simulink model " PV_PEM_direct"  (R2026a)
settings: Solver=VariableStepAuto  StopTime=sim_t
values from neighbouring files (symbols this model uses):
  Active_Area = 17.64    [ PV_PEM_direct.m]    (also in PV_PEM_direct.m)
  Irr_stair_time = (0 : Irr_stair_tsamp : sim_t)'    [ PV_PEM_direct.m]    (also in PV_PEM_direct.m)
  Irr_stair_val = interp1(Irr_time, Irr_val,  Irr_stair_time, 'linear', 0)    [ PV_PEM_direct.m]    (also in PV_PEM_direct.m)
  N = 13    [ PV_PEM_direct.m]    (also in PV_PEM_direct.m = 16)
  Ra_stack = Ra   * N    (= 0.02301)    [ PV_PEM_direct.m]    (also in PV_PEM_direct.m = 0.02832)
  Rc_stack = Rc   * N    (= 0.0065)    [ PV_PEM_direct.m]    (also in PV_PEM_direct.m = 0.008)
  Rint_stack = Rint * N    (= 0.112749)    [ PV_PEM_direct.m]    (also in PV_PEM_direct.m = 0.138768)
  sample_output_time = 60 / scale_factor    (= 0.00166666666667)    [ PV_PEM_direct.m]    (also in PV_PEM_direct.m)
  Vint_stack = Vint * N    (= 19.185933)    [ PV_PEM_direct.m]    (also in PV_PEM_direct.m = 23.613456)
libraries: fl_lib x14, nesl_utility x9, simulink x1, ee_lib x1
settings Model: Creator=hanna  LastModifiedBy=Diamantis
settings SimscapeCC: SimscapeNominalValues="[{\"value\":\"1\",\"unit\":\"A\"},{\"value\":\"1\",\"unit\":\"bar\"},{\"value\":\"1\",\"unit\":\"cm^2\"},{\"value\":\"1\",\"unit\":\"cm^3/s\"},{\"value\":\"1\",\"unit\":\"kJ/kg\"},{\"value\":\"1\",\"unit\":\"kW\"},{\"value\":\"1\",\"unit\":\"l\"},{\"value\":\"1\",\"unit\":\"N\"},{\"value\":\"1\",\"unit\":\"N*m\"},{\"value\":\"1\",\"unit\":\"V\"}]"  SimscapeLogType=none  SimscapeLogDataHistory=5000.0

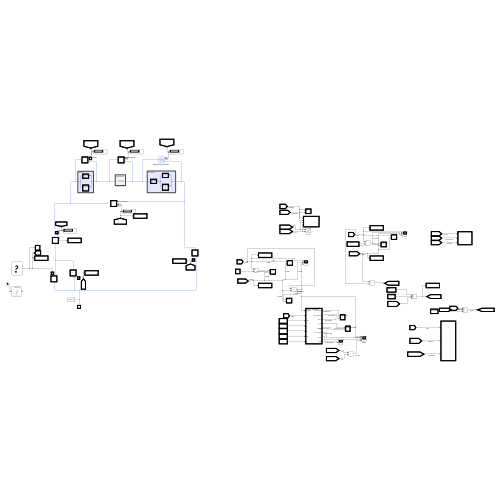
[thumbnail: Simulink's stored preview of the top-level diagram]
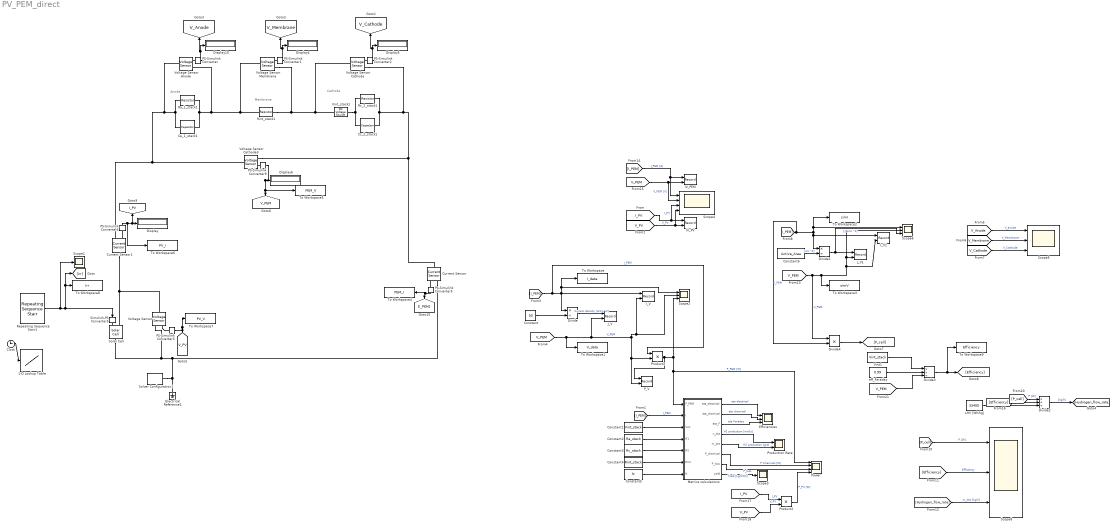
== system  PV_PEM_direct ==
  note: Membrane
  note: Cathode
  note: Anode
  1-D Lookup Table : Lookup_n-D  NumberOfTableDimensions=1  BreakpointsForDimension1=Irr_stair_time  Table=Irr_stair_val  InternalRulePriority=Speed  RndMeth=Simplest
  Ca_1_stack1 : fl_lib/Electrical/Electrical Elements/Capacitor  c=Ca_stack F  r=1e-6 Ohm  g=0 1/Ohm  i_specify=off  i_priority=None  i=0 A  i_nominal_specify=off  i_nominal_value=1  i_nominal_unit=A  v_specify=off  v_priority=None  v=0 V  v_nominal_specify=off  v_nominal_value=1  v_nominal_unit=V  vc_specify=off  vc_priority=High  vc=0 V  vc_nominal_specify=off  vc_nominal_value=1  vc_nominal_unit=V
  Cc_2_stack1 : fl_lib/Electrical/Electrical Elements/Capacitor  c=Cc_stack F  r=1e-6 Ohm  g=0 1/Ohm  i_specify=off  i_priority=None  i=0 A  i_nominal_specify=off  i_nominal_value=1  i_nominal_unit=A  v_specify=off  v_priority=None  v=0 V  v_nominal_specify=off  v_nominal_value=1  v_nominal_unit=V  vc_specify=off  vc_priority=High  vc=0 V  vc_nominal_specify=off  vc_nominal_value=1  vc_nominal_unit=V
  Clock : Clock
  Constant : Constant  Value=50
  Constant1 : Constant  Value=Vint_stack
  Constant2 : Constant  Value=Ra_stack
  Constant3 : Constant  Value=Rc_stack
  Constant4 : Constant  Value=Rint_stack
  Constant5 : Constant  Value=N
  Constant6 : Constant  Value=Active_Area
  Current Sensor : fl_lib/Electrical/Electrical Sensors/Current Sensor
  Current Sensor1 : fl_lib/Electrical/Electrical Sensors/Current Sensor
  Display{,4..6,10} (5 alike) : Display
  Divide : Product  Inputs=*/
  Divide1 : Product  Inputs=*/
  Divide2 : Product  Inputs=**/
  Divide3 : Product  Inputs=**/
  Divide4 : Product  Inputs=**
  Efficiencies : Scope  NumInputPorts=3
      settings: ActiveDisplayYMinimum=-1  ActiveDisplayYMaximum=1  DataLoggingVariableName=ScopeData5
  Electrical Reference1 : fl_lib/Electrical/Electrical Elements/Electrical Reference
  IV_PEM : Record  NumPorts=2.0  FileSettingsInternal="{\"entries\":[{\"content\":{\"excelSettings\":{\"content\":{},\"type\":\"Streamout.ExcelSettings\"},\"parquetSettings\":{\"content\":{},\"type\":\"Streamout.ParquetSettings\"}},\"type\":\"Streamout.FileSettingStorage\",\"uuid\":\"\"}],\"packageUris\":[\"http:\\/\\/schema.mathworks.com\\/mf0\\/streamout_blocks\\/R2020a\"],\"version\":\"1.0\"}"  FrameSettings=[0, 0]  Layout=[1 1]  SignalsInternal="{\"entries\":[{\"content\":{\"signals\":[{\"content\":{\"blockPath\":[],\"dimensions\":[1],\"domain\":\"\",\"lineColor\":\"#edb120\",\"lineWidth\":2,\"port\":1,\"signalID\":1,\"signalName\":\"I_PEM [A]\"},\"type\":\"RecordBlkView.Signal\",\"uuid\":\"\"},{\"content\":{\"blockPath\":[],\"dimensions\":[1],\"domain\":\"\",\"lineColor\":\"#7e2f8e\",\"lineWidth\":2,\"port\":2,\"signalID\":2,\"signalName\":\"V_PEM [V]\"},\"type\":\"RecordBlkView.Signal\",\"uuid\":\"\"}]},\"type\":\"RecordBlkView.InputSignals\",\"uuid\":\"\"}],\"packageUris\":[\"http:\\/\\/schema.mathworks.com\\/mf0\\/streamout_blocks\\/R2020a\"],\"version\":\"1.0\"}"  VisualizationBindings="{\"xyplotplugin\":{\"info\":[{\"series\":[],\"subplotID\":1}]}}"  CompatibilityTag=XY
  IV_PV : Record  NumPorts=2.0  FileSettingsInternal="{\"entries\":[{\"content\":{\"excelSettings\":{\"content\":{},\"type\":\"Streamout.ExcelSettings\"},\"parquetSettings\":{\"content\":{},\"type\":\"Streamout.ParquetSettings\"}},\"type\":\"Streamout.FileSettingStorage\",\"uuid\":\"\"}],\"packageUris\":[\"http:\\/\\/schema.mathworks.com\\/mf0\\/streamout_blocks\\/R2020a\"],\"version\":\"1.0\"}"  FrameSettings=[0, 0]  Layout=[1 1]  SignalsInternal="{\"entries\":[{\"content\":{\"signals\":[{\"content\":{\"blockPath\":[],\"dimensions\":[1],\"domain\":\"\",\"lineColor\":\"#a2142f\",\"plots\":[ 1 ],\"port\":1,\"signalID\":1,\"signalName\":\"I_PV\"},\"type\":\"RecordBlkView.Signal\",\"uuid\":\"\"},{\"content\":{\"blockPath\":[],\"dimensions\":[1],\"domain\":\"\",\"lineColor\":\"#139fff\",\"plots\":[ 1 ],\"port\":2,\"signalID\":2,\"signalName\":\"V_PV\"},\"type\":\"RecordBlkView.Signal\",\"uuid\":\"\"}]},\"type\":\"RecordBlkView.InputSignals\",\"uuid\":\"\"}],\"packageUris\":[\"http:\\/\\/schema.mathworks.com\\/mf0\\/streamout_blocks\\/R2020a\"],\"version\":\"1.0\"}"  VisualizationBindings="{\"xyplotplugin\":{\"info\":[{\"series\":[{\"bindingParametersList\":[{\"parameter\":\"X-Axis\",\"signalID\":1,\"signalName\":\"I_PV\"},{\"parameter\":\"Y-Axis\",\"signalID\":2,\"signalName\":\"V_PV\"}],\"seriesID\":0}],\"subplotID\":1}]}}"  CompatibilityTag=XY
  I_V : Record  NumPorts=2.0  FileSettingsInternal="{\"entries\":[{\"content\":{\"excelSettings\":{\"content\":{},\"type\":\"Streamout.ExcelSettings\"},\"parquetSettings\":{\"content\":{},\"type\":\"Streamout.ParquetSettings\"}},\"type\":\"Streamout.FileSettingStorage\",\"uuid\":\"\"}],\"packageUris\":[\"http:\\/\\/schema.mathworks.com\\/mf0\\/streamout_blocks\\/R2020a\"],\"version\":\"1.0\"}"  FrameSettings=[0, 0]  Layout=[1 1]  SignalsInternal="{\"entries\":[{\"content\":{\"signals\":[{\"content\":{\"blockPath\":[],\"dimensions\":[1],\"domain\":\"\",\"lineColor\":\"#a2142f\",\"lineWidth\":2,\"port\":1,\"signalID\":1,\"signalName\":\"I_PEM\"},\"type\":\"RecordBlkView.Signal\",\"uuid\":\"\"},{\"content\":{\"blockPath\":[],\"dimensions\":[1],\"domain\":\"\",\"lineColor\":\"#139fff\",\"lineWidth\":2,\"port\":2,\"signalID\":2,\"signalName\":\"V_PEM\"},\"type\":\"RecordBlkView.Signal\",\"uuid\":\"\"}]},\"type\":\"RecordBlkView.InputSignals\",\"uuid\":\"\"}],\"packageUris\":[\"http:\\/\\/schema.mathworks.com\\/mf0\\/streamout_blocks\\/R2020a\"],\"version\":\"1.0\"}"  VisualizationBindings="{\"xyplotplugin\":{\"info\":[{\"series\":[],\"subplotID\":1}]}}"  CompatibilityTag=XY
  I_V1 : Record  NumPorts=2.0  FileSettingsInternal="{\"entries\":[{\"content\":{\"excelSettings\":{\"content\":{},\"type\":\"Streamout.ExcelSettings\"},\"parquetSettings\":{\"content\":{},\"type\":\"Streamout.ParquetSettings\"}},\"type\":\"Streamout.FileSettingStorage\",\"uuid\":\"\"}],\"packageUris\":[\"http:\\/\\/schema.mathworks.com\\/mf0\\/streamout_blocks\\/R2020a\"],\"version\":\"1.0\"}"  FrameSettings=[0, 0]  Layout=[1 1]  SignalsInternal="{\"entries\":[{\"content\":{\"signals\":[{\"content\":{\"blockPath\":[],\"dimensions\":[1],\"domain\":\"\",\"lineColor\":\"#ff6929\",\"lineWidth\":2,\"port\":1,\"signalID\":1,\"signalName\":\"I_PEM\"},\"type\":\"RecordBlkView.Signal\",\"uuid\":\"\"},{\"content\":{\"blockPath\":[],\"dimensions\":[1],\"domain\":\"\",\"lineColor\":\"#b746ff\",\"lineWidth\":2,\"port\":2,\"signalID\":2,\"signalName\":\"V_PEM\"},\"type\":\"RecordBlkView.Signal\",\"uuid\":\"\"}]},\"type\":\"RecordBlkView.InputSignals\",\"uuid\":\"\"}],\"packageUris\":[\"http:\\/\\/schema.mathworks.com\\/mf0\\/streamout_blocks\\/R2020a\"],\"version\":\"1.0\"}"  VisualizationBindings="{\"xyplotplugin\":{\"info\":[{\"series\":[],\"subplotID\":1}]}}"  CompatibilityTag=XY
  J_V : Record  NumPorts=2.0  FileSettingsInternal="{\"entries\":[{\"content\":{\"excelSettings\":{\"content\":{},\"type\":\"Streamout.ExcelSettings\"},\"parquetSettings\":{\"content\":{},\"type\":\"Streamout.ParquetSettings\"}},\"type\":\"Streamout.FileSettingStorage\",\"uuid\":\"\"}],\"packageUris\":[\"http:\\/\\/schema.mathworks.com\\/mf0\\/streamout_blocks\\/R2020a\"],\"version\":\"1.0\"}"  FrameSettings=[0, 0]  Layout=[1 1]  SignalsInternal="{\"entries\":[{\"content\":{\"signals\":[{\"content\":{\"blockPath\":[],\"dimensions\":[1],\"domain\":\"\",\"lineColor\":\"#64d413\",\"lineWidth\":2,\"port\":1,\"signalID\":1,\"signalName\":\"Current density [A\\/cm^2]\"},\"type\":\"RecordBlkView.Signal\",\"uuid\":\"\"},{\"content\":{\"blockPath\":[],\"dimensions\":[1],\"domain\":\"\",\"lineColor\":\"#ff13a6\",\"lineWidth\":2,\"port\":2,\"signalID\":2,\"signalName\":\"V_PEM\"},\"type\":\"RecordBlkView.Signal\",\"uuid\":\"\"}]},\"type\":\"RecordBlkView.InputSignals\",\"uuid\":\"\"}],\"packageUris\":[\"http:\\/\\/schema.mathworks.com\\/mf0\\/streamout_blocks\\/R2020a\"],\"version\":\"1.0\"}"  VisualizationBindings="{\"xyplotplugin\":{\"info\":[{\"series\":[],\"subplotID\":1}]}}"  CompatibilityTag=XY
  J_V1 : Record  NumPorts=2.0  FileSettingsInternal="{\"entries\":[{\"content\":{\"excelSettings\":{\"content\":{},\"type\":\"Streamout.ExcelSettings\"},\"parquetSettings\":{\"content\":{},\"type\":\"Streamout.ParquetSettings\"}},\"type\":\"Streamout.FileSettingStorage\",\"uuid\":\"\"}],\"packageUris\":[\"http:\\/\\/schema.mathworks.com\\/mf0\\/streamout_blocks\\/R2020a\"],\"version\":\"1.0\"}"  FrameSettings=[0, 0]  Layout=[1 1]  SignalsInternal="{\"entries\":[{\"content\":{\"signals\":[{\"content\":{\"blockPath\":[],\"dimensions\":[1],\"domain\":\"\",\"lineColor\":\"#fe330a\",\"lineWidth\":2,\"port\":1,\"signalID\":1,\"signalName\":\"J [A\\/cm^2]\"},\"type\":\"RecordBlkView.Signal\",\"uuid\":\"\"},{\"content\":{\"blockPath\":[],\"dimensions\":[1],\"domain\":\"\",\"lineColor\":\"#22b573\",\"lineWidth\":2,\"port\":2,\"signalID\":2,\"signalName\":\"V_PEM\"},\"type\":\"RecordBlkView.Signal\",\"uuid\":\"\"}]},\"type\":\"RecordBlkView.InputSignals\",\"uuid\":\"\"}],\"packageUris\":[\"http:\\/\\/schema.mathworks.com\\/mf0\\/streamout_blocks\\/R2020a\"],\"version\":\"1.0\"}"  VisualizationBindings="{\"xyplotplugin\":{\"info\":[{\"series\":[],\"subplotID\":1}]}}"  CompatibilityTag=XY
  LHV [Wh/kg] : Constant  Value=33400
  Metrics calculations : MATLAB Function  TreatAsAtomicUnit=on
  PS-Simulink Converter{,1..2,5,9} (5 alike) : nesl_utility/PS-Simulink Converter  PhysicalDomain=network_engine_domain  SubClassName=ps_output  LeftPortType=input  RightPortType=output  PseudoPeriodic=off  Frequencies=[]  VectorFormat=inherit  Unit=inherit  AffineConversion=off
  PS-Simulink Converter3 : nesl_utility/PS-Simulink Converter  PhysicalDomain=network_engine_domain  SubClassName=ps_output  LeftPortType=input  RightPortType=output  PseudoPeriodic=off  Frequencies=[]  VectorFormat=1-D array  Unit=V  AffineConversion=off
  PS-Simulink Converter4 : nesl_utility/PS-Simulink Converter  PhysicalDomain=network_engine_domain  SubClassName=ps_output  LeftPortType=input  RightPortType=output  PseudoPeriodic=off  Frequencies=[]  VectorFormat=1-D array  Unit=A  AffineConversion=off
  P_V : Record  NumPorts=2.0  FileSettingsInternal="{\"entries\":[{\"content\":{\"excelSettings\":{\"content\":{},\"type\":\"Streamout.ExcelSettings\"},\"parquetSettings\":{\"content\":{},\"type\":\"Streamout.ParquetSettings\"}},\"type\":\"Streamout.FileSettingStorage\",\"uuid\":\"\"}],\"packageUris\":[\"http:\\/\\/schema.mathworks.com\\/mf0\\/streamout_blocks\\/R2020a\"],\"version\":\"1.0\"}"  FrameSettings=[0, 0]  Layout=[1 1]  SignalsInternal="{\"entries\":[{\"content\":{\"signals\":[{\"content\":{\"blockPath\":[],\"dimensions\":[1],\"domain\":\"\",\"lineColor\":\"#0072bd\",\"lineWidth\":2,\"port\":1,\"signalID\":1,\"signalName\":\"P_PEM [W]\"},\"type\":\"RecordBlkView.Signal\",\"uuid\":\"\"},{\"content\":{\"blockPath\":[],\"dimensions\":[1],\"domain\":\"\",\"lineColor\":\"#d95319\",\"lineWidth\":2,\"port\":2,\"signalID\":2,\"signalName\":\"V_PEM\"},\"type\":\"RecordBlkView.Signal\",\"uuid\":\"\"}]},\"type\":\"RecordBlkView.InputSignals\",\"uuid\":\"\"}],\"packageUris\":[\"http:\\/\\/schema.mathworks.com\\/mf0\\/streamout_blocks\\/R2020a\"],\"version\":\"1.0\"}"  VisualizationBindings="{\"xyplotplugin\":{\"info\":[{\"series\":[],\"subplotID\":1}]}}"  CompatibilityTag=XY
  Power : Scope  NumInputPorts=4
      settings: ActiveDisplayYMinimum=-1  ActiveDisplayYMaximum=1  DataLoggingVariableName=ScopeData6
  Product1 : Product
  Product2 : Product
  Production Rate : Scope  NumInputPorts=2
      settings: ActiveDisplayYMinimum=-6.6507662971533038E-5  ActiveDisplayYMaximum=0.00059856896673107221  DataLoggingVariableName=ScopeData7
  Ra_1_stack1 : fl_lib/Electrical/Electrical Elements/Resistor  R=Ra_stack Ohm  i_specify=off  i_priority=None  i=0 A  i_nominal_specify=off  i_nominal_value=1  i_nominal_unit=A  v_specify=off  v_priority=None  v=0 V  v_nominal_specify=off  v_nominal_value=1  v_nominal_unit=V
  Rc_2_stack1 : fl_lib/Electrical/Electrical Elements/Resistor  R=Rc_stack Ohm  i_specify=off  i_priority=None  i=0 A  i_nominal_specify=off  i_nominal_value=1  i_nominal_unit=A  v_specify=off  v_priority=None  v=0 V  v_nominal_specify=off  v_nominal_value=1  v_nominal_unit=V
  Repeating Sequence Stair1 : simulink/Sources/Repeating Sequence Stair  OutValues=Irr_stair_val  tsamp=Irr_stair_tsamp  OutMin=[]  OutMax=[]  OutDataTypeStr=double  OutputDataTypeScalingMode=double  OutDataType=fixdt(0,8)  ConRadixGroup=Best Precision: Vector-wise  OutScaling=2^-12
  Rint_stack1 : fl_lib/Electrical/Electrical Elements/Resistor  R=Rint_stack Ohm  i_specify=off  i_priority=None  i=0 A  i_nominal_specify=off  i_nominal_value=1  i_nominal_unit=A  v_specify=off  v_priority=None  v=0 V  v_nominal_specify=off  v_nominal_value=1  v_nominal_unit=V
  Scope1 : Scope
      settings: ActiveDisplayYMinimum=-124.99999999999997  ActiveDisplayYMaximum=1125
  Scope{2,5..6,8} (4 alike) : Scope  NumInputPorts=3
      Scope2 settings: ActiveDisplayYMinimum=-2.2100954998449684  ActiveDisplayYMaximum=19.79179103183268  DataLoggingVariableName=ScopeData2
      Scope5 settings: ActiveDisplayYMinimum=-0.025574999999999994  ActiveDisplayYMaximum=0.23017500000000002  DataLoggingVariableName=ScopeData8
      Scope6 settings: ActiveDisplayYMinimum=2.1952046709351865  ActiveDisplayYMaximum=2.2345014292442293  DataLoggingVariableName=ScopeData10
      Scope8 settings: ActiveDisplayString=3  ActiveDisplayYMinimum=-0.0016083601949654486  ActiveDisplayYMaximum=0.014332465135728535
  Scope3 : Scope
      settings: ActiveDisplayYMinimum=-1  ActiveDisplayYMaximum=1  DataLoggingVariableName=ScopeData3
  Scope4 : Scope  NumInputPorts=4
      settings: ActiveDisplayYMinimum=-6.1277884950416563  ActiveDisplayYMaximum=54.606123205001168  DataLoggingVariableName=ScopeData9
  Simulink-PS Converter5 : nesl_utility/Simulink-PS Converter  PhysicalDomain=network_engine_domain  SubClassName=ps_input  LeftPortType=input  RightPortType=output  PseudoPeriodic=off  Frequencies=[]  NoiseDistribution=none  NoiseParameters=[]  Unit=1  AffineConversion=off  FilteringAndDerivatives=provide  SimscapeFilterOrder=1  InputFilterTimeConstant=0.001  UdotUserProvided=0
  Solar Cell : ee_lib/Sources/Solar Cell  PartSpecification="{\"CollectionId\":\"SimscapeElectrical\",\"CollectionVersion\":\"1.0.0\",\"DatasetId\":\"Amerisolar|AS_6M30_HC_320W|simscape.electrical.solarCell\",\"DisplayName\":\"Amerisolar:AS_6M30_HC_320W\"}"  prm=3  Isc=10.14 % Datasheet derived A  Voc=0.67 % Datasheet derived V  Is=3.24823447983853e-07 % Datasheet derived A  Is2=9.37081970792037e-10 % Datasheet derived A  Iph=10.140005507508 % Datasheet derived A  Ir0=1000 % Datasheet derived W/m^2  ec=1.51118472243322 % Datasheet derived  N2=2.60259908345858 % Datasheet derived  Rs=1.94548269975201e-05 % Datasheet derived Ohm  Rp=682.95993142779 % Datasheet derived Ohm  N_series=Ns_cell % Datasheet derived  N_parallel=Np_cell % Datasheet derived  TIPH1=0.000499942933005141 % Datasheet derived 1/K  EG=1.12 % Datasheet derived eV  TXIS1=4.23641510120988 % Datasheet derived  TXIS2=16.2689137700667 % Datasheet derived  TRS1=0.243341028305912 % Datasheet derived  TRP1=0 % Parameter not set  Tmeas=25 % Datasheet derived degC  TFIXED=25 % Datasheet derived degC  thermal_mass=100 % Parameter not set J/K  initial_temperature=25 degC
      settings: AttributesFormatString=Amerisolar:AS_6M30_HC_320W
  Solver Configuration1 : nesl_utility/Solver Configuration  PhysicalDomain=network_engine_domain  SubClassName=solver  LeftPortType=input  RightPortType=generic  Tones=[]  Harmonics=[]  SimulateNoise=off  Profile=off  UseLocalSampling=off  EnableSwitchedLinearOptims=on  FrequencyDomain=off  UseCCode=off  RelTol=0.001  AbsTol=0.001  MinStep=1e-09  ToWorkspace=off  RevertToSquareIcSolve=off  NumHomotopyIterations=100  PhasorMode=off  PhasorModeNumHarmonics=1  ConsistencySolver=NEWTON_XTOL_AFTER_FTOL  CanonicalOrdering=UNORDERED  OptimizeIntermediates=UNOPTIMIZED  IndexReductionMethod=DerivativeReplacement  DoDC=off  ResidualTolerance=1e-09  ConsistencyTolSource=GLOBAL  ConsistencyAbsTol=0.001  ConsistencyRelTol=0.001  ConsistencyTolFactor=0.001  UseLocalSolver=off  LocalSolverChoice=NE_BACKWARD_EULER_ADVANCER  ResolveIndetEquations=on  FunctionEvalNumThread=1  LocalSolverSampleTime=0.001  DoFixedCost=off  MaxNonlinIter=3  MaxModeIter=2  ComputeImpulses=off  ImpulseIterations=2  LinearAlgebra=auto  LinearAlgebraNumThread=0  EquationFormulation=NE_TIME_EF  DelaysMemoryBudget=1024  AutomaticFiltering=on  FilteringTimeConstant=0.001  PartitionStorageMethod=AS_NEEDED  PartitionMemoryBudget=1024  PartitionMethod=ROBUST  MultibodyUseLocalSolver=off  MultibodyLocalSolverChoice=ODE1  MultibodyLocalSolverSampleTime=0.001
  To Workspace : ToWorkspace  VariableName=I_data  SaveFormat=Timeseries  SampleTime=-1
  To Workspace1 : ToWorkspace  VariableName=V_data  SaveFormat=Timeseries  SampleTime=-1
  To Workspace2 : ToWorkspace  VariableName=simI  SaveFormat=Timeseries  SampleTime=0.1
  To Workspace3 : ToWorkspace  VariableName=simV  SaveFormat=Timeseries  SampleTime=0.1
  To Workspace4 : ToWorkspace  VariableName=PEM_I  SaveFormat=Timeseries  SampleTime=sample_output_time
  To Workspace5 : ToWorkspace  VariableName=PEM_V  SaveFormat=Timeseries  SampleTime=sample_output_time
  To Workspace6 : ToWorkspace  VariableName=PV_I  SaveFormat=Timeseries  SampleTime=sample_output_time
  To Workspace7 : ToWorkspace  VariableName=PV_V  SaveFormat=Timeseries  SampleTime=sample_output_time
  To Workspace8 : ToWorkspace  VariableName=Irr  SaveFormat=Timeseries  SampleTime=sample_output_time
  To Workspace9 : ToWorkspace  VariableName=Efficiency  SaveFormat=Timeseries  SampleTime=-1
  Vint1 : Constant  Value=Vint_stack
  Vint_stack1 : fl_lib/Electrical/Electrical Sources/DC Voltage Source  v0=Vint_stack V
  Voltage Sensor : fl_lib/Electrical/Electrical Sensors/Voltage Sensor
  Voltage Sensor Anode : fl_lib/Electrical/Electrical Sensors/Voltage Sensor
  Voltage Sensor Cathode : fl_lib/Electrical/Electrical Sensors/Voltage Sensor
  Voltage Sensor Cathode3 : fl_lib/Electrical/Electrical Sensors/Voltage Sensor
  Voltage Sensor Membrane : fl_lib/Electrical/Electrical Sensors/Voltage Sensor
  eff_Faraday : Constant  Value=0.99
  tag scope: I_PV=global, V_Anode=global, V_Cathode=global, V_Membrane=global, V_PEM=global, V_PV=global
  wires:
  Repeating Sequence Stair1/1 -> Simulink-PS Converter5/1, To Workspace8/1, [Irr], Scope1/1
  Clock/1 -> 1-D Lookup Table/1
  Constant/1 -> Divide/2
  [V_PEM] -> I_V/2, Scope2/2, Product1/2, P_V/2, J_V/2, To Workspace1/1  "V_PEM"
  [I_PEM] -> I_V/1, Divide/1, To Workspace/1, Scope2/1, Product1/1  "I_PEM"
  Divide/1 -> J_V/1  "Current density [A/cm^2]"
  Product1/1 -> P_V/1, Metrics calculations/1(P_PEM), Power/1, Scope2/3  "P_PEM [W]"
  [I_PEM] -> Metrics calculations/2(I)  "I_PEM"
  Metrics calculations/5(m_dot) -> Production Rate/2  "H2 production [g/s]"
  Constant4/1 -> Metrics calculations/6(Rint)
  Constant3/1 -> Metrics calculations/5(R2)
  Constant2/1 -> Metrics calculations/4(R1)
  Constant1/1 -> Metrics calculations/3(Vint)
  [V_PV] -> Scope4/4, IV_PV/2  "V_PV"
  [I_PV] -> Scope4/3, IV_PV/1  "I_PV"
  [I_PV] -> Product2/1  "I_PV"
  [V_PV] -> Product2/2  "V_PV"
  Product2/1 -> Power/4  "P_PV [W]"
  Metrics calculations/6(P_chemical) -> Power/2  "P Chemical [W]"
  Metrics calculations/1(eta_electrical) -> Efficiencies/1  "eta electrical"
  Metrics calculations/2(eta_chemical) -> Efficiencies/2  "eta chemical"
  Metrics calculations/3(eta_F) -> Efficiencies/3  "eta Faraday"
  Metrics calculations/4(n_dot) -> Production Rate/1  "H2 production [mol/s]"
  Metrics calculations/7(P_loss) -> Power/3  "P_loss"
  Metrics calculations/8(yield) -> Scope3/1  "Yield [kg/kWh]"
  Constant5/1 -> Metrics calculations/7(N)
  [V_Membrane] -> Scope5/2  "V_Membrane"
  Divide3/1 -> To Workspace9/1, [Efficiency]
  [Efficiency] -> Scope8/2  "Efficiency"
  [I_PEM] -> Scope4/1, IV_PEM/1  "I_PEM [A]"
  [V_PEM] -> Scope4/2, IV_PEM/2  "V_PEM [V]"
  Vint1/1 -> Divide3/1
  Divide4/1 -> [P_cell]
  [I_PEM] -> Scope6/1, To Workspace2/1, Divide1/1, I_V1/1, Divide4/2  "I_PEM"
  Divide1/1 -> Scope6/3, J_V1/1  "J [A/cm^2]"
  [Efficiency] -> Divide2/2
  [Hydrogen_flow_rate] -> Scope8/3  "m_dot [kg/h]"
  [V_Anode] -> Scope5/1  "V_anode"
  [P_cell] -> Scope8/1  "P [W]"
  LHV [Wh/kg]/1 -> Divide2/3
  [P_cell] -> Divide2/1  "P [W]"
  [V_PEM] -> Divide4/1, To Workspace3/1, Scope6/2, J_V1/2, I_V1/2  "V_PEM"
  eff_Faraday/1 -> Divide3/2
  [V_Cathode] -> Scope5/3  "V_Cathode"
  Divide2/1 -> [Hydrogen_flow_rate]  "[kg/h]"
  Constant6/1 -> Divide1/2  "[cm^2]"
  [V_PEM] -> Divide3/3
  PS-Simulink Converter1/1 -> [V_Membrane], Display4/1
  PS-Simulink Converter9/1 -> To Workspace5/1, [V_PEM], Display6/1
  PS-Simulink Converter/1 -> [V_Anode], Display10/1
  PS-Simulink Converter2/1 -> [V_Cathode], Display5/1
  PS-Simulink Converter4/1 -> To Workspace6/1, [I_PV], Display/1
  PS-Simulink Converter5/1 -> To Workspace4/1, [I_PEM]
  PS-Simulink Converter3/1 -> To Workspace7/1, [V_PV]
  connections:
  Solver Configuration1/RConn1 -- Voltage Sensor/RConn2 -- Solar Cell/RConn1 -- Current Sensor/RConn2 -- Electrical Reference1/LConn1
  Simulink-PS Converter5/RConn1 -- Solar Cell/LConn1
  Current Sensor1/LConn1 -- Voltage Sensor/LConn1 -- Solar Cell/LConn2
  Voltage Sensor Anode/RConn2 -- Ra_1_stack1/RConn1 -- Ca_1_stack1/RConn1 -- Rint_stack1/LConn1 -- Voltage Sensor Membrane/LConn1
  Voltage Sensor Anode/LConn1 -- Ca_1_stack1/LConn1 -- Ra_1_stack1/LConn1 -- Current Sensor1/RConn2 -- Voltage Sensor Cathode3/LConn1
  Voltage Sensor Membrane/RConn2 -- Voltage Sensor Cathode/LConn1 -- Vint_stack1/LConn1 -- Rint_stack1/RConn1
  Cc_2_stack1/RConn1 -- Rc_2_stack1/RConn1 -- Current Sensor/LConn1 -- Voltage Sensor Cathode3/RConn2 -- Voltage Sensor Cathode/RConn2
  Cc_2_stack1/LConn1 -- Vint_stack1/RConn1 -- Rc_2_stack1/LConn1
  Voltage Sensor Cathode3/RConn1 -- PS-Simulink Converter9/LConn1
  Voltage Sensor Membrane/RConn1 -- PS-Simulink Converter1/LConn1
  Voltage Sensor Cathode/RConn1 -- PS-Simulink Converter2/LConn1
  Voltage Sensor Anode/RConn1 -- PS-Simulink Converter/LConn1
  Current Sensor1/RConn1 -- PS-Simulink Converter4/LConn1
  PS-Simulink Converter5/LConn1 -- Current Sensor/RConn1
  PS-Simulink Converter3/LConn1 -- Voltage Sensor/RConn1

== matlab function  PV_PEM_direct/Metrics calculations ==
  data: P_PEM input; I input; Vint input; R1 input; R2 input; Rint input; eta_electrical output; eta_chemical output; eta_F output; n_dot output; m_dot output; P_chemical output; P_loss output; yield output; N input

function [eta_electrical, eta_chemical, eta_F,n_dot, m_dot,P_chemical, P_loss, yield]   = pem_eff( P_PEM, I,Vint, R1, R2, Rint, N)

Rsum = R1 + R2 + Rint;
eta_electrical = (I*Vint) / (I*Vint + I^2 * Rsum); % Guilbert et al. = eta electrical = eta_PV_H2

area = 0.005; %[m^2]
i_el = I / area; %current density [A/m^2]
eta_F_percent = 96.5 * exp(0.09 / i_el - 75.5 / i_el^2);  %Yodwong et al.
eta_F = eta_F_percent/100; 
F_constant = 96485.33; %[s*A/mol]

n_dot = eta_F*I*N/(2*F_constant); %[mol/s]

HHV = 286000; %[J/mol]
P_chemical = n_dot * HHV; %[W]

molar_mass = 2.016; %[g/mol]
m_dot = n_dot * molar_mass; % [g/s]
m_dot_kg_h = m_dot * 3.6; %[kg/h]

eta_chemical = P_chemical/P_PEM; 

P_loss = P_PEM - P_chemical; 

yield = m_dot_kg_h/(P_PEM/1000); %[kg/Wh]


end
%Faradaic efficiency = 1 which means that the resulting efficiency and
%hydrogen production is the upper limit
%change it later to variables being saved in a way that they can be used in the function and onl need I input
% eta equation from Guilbert et al.
